simulink model "fp_sum"  (Simulink 7.6)
settings: Solver=FixedStepDiscrete  StartTime=0.0  StopTime=1  FixedStep=1  RelTol=1e-3
settings Model: Creator=jordan  LastModifiedBy=jordan
settings DataIOCC: LimitDataPoints=off  SaveOutput=off  SignalLogging=off  DSMLogging=off  SaveTime=off
settings OptimizationCC: BlockReduction=off  ConditionallyExecuteInputs=off

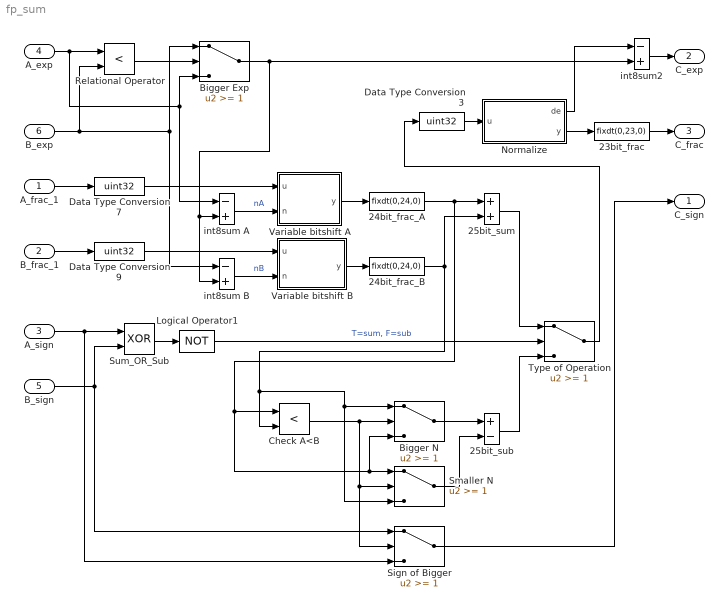
== system fp_sum ==
  A_frac_1 : Inport  OutDataTypeStr=fixdt(0,24,0)
  B_frac_1 : Inport  Port=2  OutDataTypeStr=fixdt(0,24,0)
  A_sign : Inport  Port=3  OutDataTypeStr=boolean
  A_exp : Inport  Port=4  OutDataTypeStr=uint8
  B_sign : Inport  Port=5  OutDataTypeStr=boolean
  B_exp : Inport  Port=6  OutDataTypeStr=uint8
  23bit_frac : DataTypeConversion  OutDataTypeStr=fixdt(0,23,0)
  24bit_frac_A : DataTypeConversion  OutDataTypeStr=fixdt(0,24,0)
  24bit_frac_B : DataTypeConversion  OutDataTypeStr=fixdt(0,24,0)
  25bit_sub : Sum  Inputs=+-  OutDataTypeStr=fixdt(0,25,0)  RndMeth=Nearest  SaturateOnIntegerOverflow=on
  25bit_sum : Sum  OutDataTypeStr=fixdt(0,25,0)  RndMeth=Nearest  SaturateOnIntegerOverflow=on
  Bigger Exp : Switch  Threshold=1  RndMeth=Nearest
  Bigger N : Switch  Threshold=1
  Check A<B : RelationalOperator  Operator=<  OutDataTypeStr=boolean
  Data Type Conversion3 : DataTypeConversion  OutDataTypeStr=uint32
  Data Type Conversion7 : DataTypeConversion  OutDataTypeStr=uint32
  Data Type Conversion9 : DataTypeConversion  OutDataTypeStr=uint32
  Logical Operator1 : Logic  Operator=NOT  AllPortsSameDT=off  OutDataTypeStr=boolean
  Normalize : Stateflow chart  TreatAsAtomicUnit=on
  Relational Operator : RelationalOperator  Operator=<  OutDataTypeStr=boolean
  Sign of Bigger : Switch  Threshold=1
  Smaller N : Switch  Threshold=1
  Sum_OR_Sub : Logic  Operator=XOR  AllPortsSameDT=off  OutDataTypeStr=boolean
  Type of Operation : Switch  Threshold=1
  Variable bitshift A : Stateflow chart  TreatAsAtomicUnit=on
  Variable bitshift B : Stateflow chart  TreatAsAtomicUnit=on
  int8sum A : Sum  Inputs=-+  OutDataTypeStr=int8  RndMeth=Nearest  SaturateOnIntegerOverflow=on
  int8sum B : Sum  Inputs=-+  OutDataTypeStr=int8  RndMeth=Nearest  SaturateOnIntegerOverflow=on
  int8sum2 : Sum  Inputs=-+  OutDataTypeStr=uint8  RndMeth=Nearest  SaturateOnIntegerOverflow=on
  C_sign : Outport  OutDataTypeStr=boolean
  C_exp : Outport  Port=2  OutDataTypeStr=uint8
  C_frac : Outport  Port=3  OutDataTypeStr=fixdt(0,23,0)
  wires:
  A_exp/1 -> Relational Operator/1, Bigger Exp/3, int8sum A/1
  B_exp/1 -> Bigger Exp/1, int8sum B/1, Relational Operator/2
  A_frac_1/1 -> Data Type Conversion7/1
  Variable bitshift A/1(y) -> 24bit_frac_A/1
  24bit_frac_A/1 -> 25bit_sum/1, Check A<B/1, Smaller N/1, Bigger N/3
  Relational Operator/1 -> Bigger Exp/2
  Bigger Exp/1 -> int8sum2/2, int8sum A/2, int8sum B/2
  B_frac_1/1 -> Data Type Conversion9/1
  int8sum A/1 -> Variable bitshift A/2(n)  "nA"
  int8sum B/1 -> Variable bitshift B/2(n)  "nB"
  Variable bitshift B/1(y) -> 24bit_frac_B/1
  24bit_frac_B/1 -> 25bit_sum/2, Check A<B/2, Bigger N/1, Smaller N/3
  25bit_sum/1 -> Type of Operation/1
  Normalize/2(y) -> 23bit_frac/1
  Normalize/1(de) -> int8sum2/1
  Data Type Conversion3/1 -> Normalize/1(u)
  23bit_frac/1 -> C_frac/1
  Sum_OR_Sub/1 -> Logical Operator1/1
  Logical Operator1/1 -> Type of Operation/2  "T=sum, F=sub"
  Check A<B/1 -> Bigger N/2, Smaller N/2, Sign of Bigger/2
  Bigger N/1 -> 25bit_sub/1
  Smaller N/1 -> 25bit_sub/2
  25bit_sub/1 -> Type of Operation/3
  Type of Operation/1 -> Data Type Conversion3/1
  Sign of Bigger/1 -> C_sign/1
  Data Type Conversion7/1 -> Variable bitshift A/1(u)
  Data Type Conversion9/1 -> Variable bitshift B/1(u)
  A_sign/1 -> Sum_OR_Sub/1, Sign of Bigger/3
  B_sign/1 -> Sum_OR_Sub/2, Sign of Bigger/1
  int8sum2/1 -> C_exp/1

== matlab function Variable bitshift A ==
  data: u input uint32; y output uint32; n input int8
function y = bitshift(u,n)
%#eml

y = bitshift(u,-n);

== matlab function Variable bitshift B ==
  data: u input uint32; y output uint32; n input int8
function y = bitshift(u,n)
%#eml

y = bitshift(u,-n);

== matlab function Normalize ==
  data: de output double; u input uint32; y output uint32
function [de,y] = Normalize(u)
%#eml

buf=u;
p=int8(-1);
c=bitand(buf,2^24);
for ind=1:25
    if (~c)
        p=p+1;
        buf=bitshift(buf,1);
        c=bitand(buf,2^24);
    end
end
bufy = bitand(bitshift(u,p),2^23-1);
y=bufy;
de=p;
